simulink model "spart_sim_test"  (R2022a)
settings: Solver=VariableStepAuto  StartTime=0.0  StopTime=10.0  RelTol=1e-3
undefined symbols (not defined in the file or in its folder): M0, um0
libraries: SPART_Lib x3
settings Model: Creator=charl  LastModifiedBy=charl

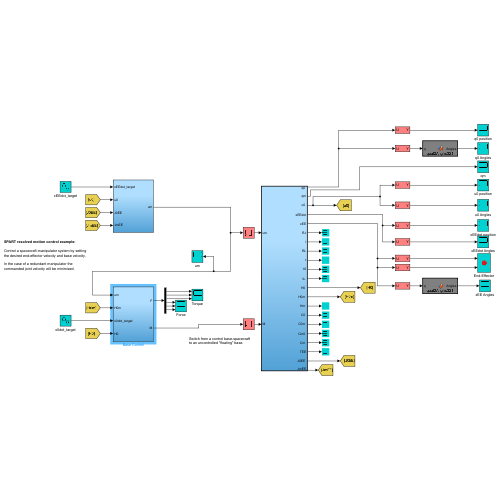
[thumbnail: Simulink's stored preview of the top-level diagram]
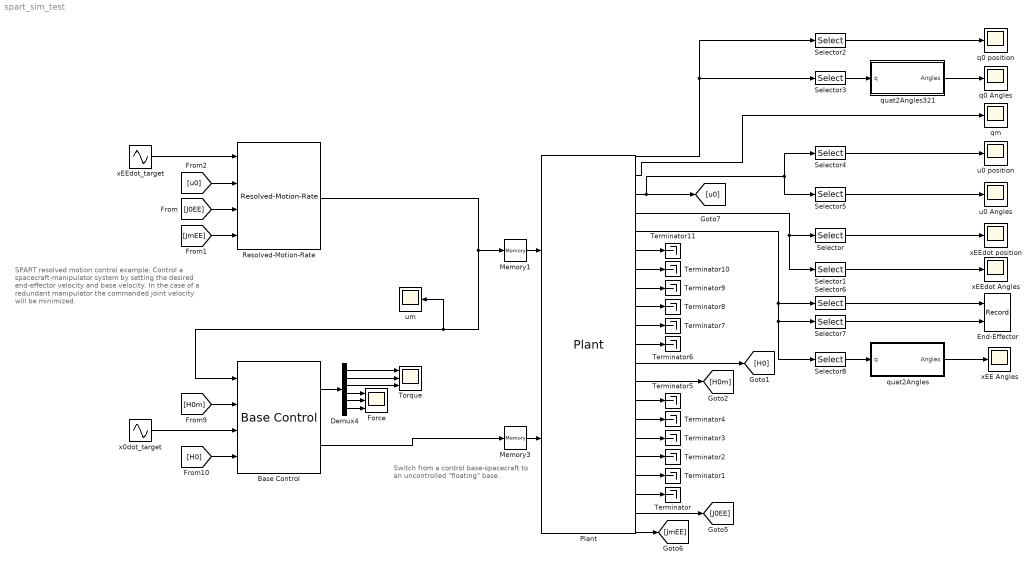
== system spart_sim_test ==
  note: SPART resolved motion control example:
      |
      | Control a spacecraft-manipulator system by setting the desired end-effector velocity and base velocity.
      |
      | In the case of a redundant manipulator the commanded joint velocity will be minimized.
  note: Switch from a control base-spacecraft to an uncontrolled "floating" base.
  Base Control : SPART_Lib/Control/Base Control  SystemSampleTime=-1  VariantActivationTime=update diagram  Latency=0  AutoFrameSizeCalculation=off
  Demux4 : Demux  Outputs=6
  End-Effector : Record  FileSettingsInternal="{\"entries\":[{\"content\":{\"excelSettings\":{\"content\":{},\"type\":\"Streamout.ExcelSettings\"}},\"type\":\"Streamout.FileSettingStorage\",\"uuid\":\"04699d78-4616-4cef-81af-d9585e3b4ee2\"}],\"packageUris\":[\"http://schema.mathworks.com/mf0/streamout_blocks/R2020a\"],\"version\":\"1.0\"}"  Layout=[1 1]  SignalsInternal="{\"entries\":[{\"content\":{\"signals\":[{\"content\":{\"blockPath\":[\"spart_sim_test/End-Effector\"],\"channel\":[],\"dimensions\":[1,1],\"domain\":\"spart_sim_test/End-Effector\",\"lineColor\":\"#a2142f\",\"plots\":[1],\"port\":1,\"sid\":[\"\"],\"signalID\":227,\"signalName\":\"Selector6\"},\"type\":\"RecordBlkView.Signal\",\"uuid\":\"8d9be762-1d05-4863-8dca-644fe018a486\"},{\"content\":{\"blockPath\":[\"spart_sim_test/End-Effector\"],\"channel\":[],\"dimensions\":[1,1],\"domain\":\"spart_sim_test/End-Effector\",\"lineColor\":\"#139fff\",\"plots\":[1],\"port\":2,\"sid\":[\"\"],\"signalID\":231,\"signalName\":\"Selector7\"},\"type\":\"RecordBlkView.Signal\",\"uuid\":\"098425a8-9d72-4562-8d53-08ba24e55e97\"}]},\"type\":\"RecordBlkView.InputSignals\",\"uuid\":\"7cb01df9-89e0-49c5-adc4-e9907efb910e\"}],\"packageUris\":[\"http://schema.mathworks.com/mf0/streamout_blocks/R2020a\"],\"version\":\"1.0\"}"  VisualizationBindings="{\"xyplotplugin\":{\"info\":[{\"series\":[{\"bindingParametersList\":[{\"parameter\":\"X-Axis\",\"signalID\":227,\"signalName\":\"Selector6\"},{\"parameter\":\"Y-Axis\",\"signalID\":231,\"signalName\":\"Selector7\"}],\"seriesID\":21343}],\"subplotID\":1}]}}"  CompatibilityTag=XY  st=-1
  Force : Scope  NumInputPorts=3
  Memory1 : Memory  InitialCondition=um0  InheritSampleTime=on
  Memory3 : Memory  InitialCondition=M0  InheritSampleTime=on
  Plant : SPART_Lib/Plant  SystemSampleTime=-1  VariantActivationTime=update diagram  Latency=0  AutoFrameSizeCalculation=off
  "Resolved-Motion-Rate " : SPART_Lib/Control/Resolved-Motion-Rate   SystemSampleTime=-1  VariantActivationTime=update diagram  Latency=0  AutoFrameSizeCalculation=off
  Selector : Selector  InputPortWidth=6  IndexOptions=Index vector (dialog)  Indices=[4:6]  OutputSizes=1
  Selector1 : Selector  InputPortWidth=6  IndexOptions=Index vector (dialog)  Indices=[1:3]  OutputSizes=1
  Selector2 : Selector  InputPortWidth=7  IndexOptions=Index vector (dialog)  Indices=[5:7]  OutputSizes=1
  Selector3 : Selector  InputPortWidth=7  IndexOptions=Index vector (dialog)  Indices=[1:4]  OutputSizes=1
  Selector4 : Selector  InputPortWidth=6  IndexOptions=Index vector (dialog)  Indices=[4:6]  OutputSizes=1
  Selector5 : Selector  InputPortWidth=6  IndexOptions=Index vector (dialog)  Indices=[1:3]  OutputSizes=1
  Selector6 : Selector  InputPortWidth=7  IndexOptions=Index vector (dialog)  Indices=[5]  OutputSizes=1
  Selector7 : Selector  InputPortWidth=7  IndexOptions=Index vector (dialog)  Indices=[6]  OutputSizes=1
  Selector8 : Selector  InputPortWidth=7  IndexOptions=Index vector (dialog)  Indices=[1:4]  OutputSizes=1
  Terminator{,1..11} (12 alike) : Terminator
  Torque : Scope  NumInputPorts=3
  q0 Angles : Scope
  "q0 position " : Scope
  qm : Scope
  quat2Angles : MATLAB Function  TreatAsAtomicUnit=on
  quat2Angles321 : MATLAB Function  TreatAsAtomicUnit=on
  u0 Angles : Scope
  u0 position : Scope
  um : Scope
  x0dot_target : Sin  Amplitude=[0;0;0.05;0;0;0]  Frequency=pi/4  SampleTime=0
  xEE Angles : Scope
  xEEdot Angles : Scope
  xEEdot position : Scope
  xEEdot_target : Sin  Amplitude=[0;0;0.1;0.05;0.05;0]  Frequency=pi/2  Phase=[0;0;0;0;pi/2;0]  SampleTime=0
  wires:
  Plant/21 -> [JmEE]
  Selector1/1 -> xEEdot Angles/1
  Plant/9 -> Terminator8/1
  Memory1/1 -> Plant/1
  Base Control/2 -> Memory3/1
  [H0] -> Base Control/4
  Memory3/1 -> Plant/2
  Plant/16 -> Terminator3/1
  quat2Angles321/1(Angles) -> q0 Angles/1
  Selector3/1 -> quat2Angles321/1(q)
  [J0EE] -> "Resolved-Motion-Rate "/3
  Plant/19 -> Terminator/1
  Selector7/1 -> End-Effector/2
  Selector6/1 -> End-Effector/1
  "Resolved-Motion-Rate "/1 -> Base Control/1, um/1, Memory1/1
  Selector4/1 -> u0 position/1
  Selector/1 -> xEEdot position/1
  Plant/1 -> Selector2/1, Selector3/1
  Plant/14 -> Terminator5/1
  Plant/11 -> Terminator6/1
  Plant/10 -> Terminator7/1
  Selector8/1 -> quat2Angles/1(q)
  Plant/8 -> Terminator9/1
  Plant/5 -> Selector6/1, Selector7/1, Selector8/1
  Selector2/1 -> "q0 position "/1
  quat2Angles/1(Angles) -> xEE Angles/1
  Plant/4 -> Selector1/1, Selector/1
  Demux4/5 -> Force/2
  Demux4/3 -> Torque/3
  Plant/7 -> Terminator10/1
  Demux4/6 -> Force/3
  Demux4/1 -> Torque/1
  Plant/15 -> Terminator4/1
  Base Control/1 -> Demux4/1
  Plant/17 -> Terminator2/1
  [u0] -> "Resolved-Motion-Rate "/2
  Plant/3 -> Selector4/1, Selector5/1, [u0]
  Demux4/4 -> Force/1
  Plant/6 -> Terminator11/1
  x0dot_target/1 -> Base Control/3
  Plant/20 -> [J0EE]
  Demux4/2 -> Torque/2
  [H0m] -> Base Control/2
  xEEdot_target/1 -> "Resolved-Motion-Rate "/1
  [JmEE] -> "Resolved-Motion-Rate "/4
  Selector5/1 -> u0 Angles/1
  Plant/12 -> [H0]
  Plant/2 -> qm/1
  Plant/13 -> [H0m]
  Plant/18 -> Terminator1/1

== matlab function spart_sim_test/quat2Angles321 ==
  data: q input; Angles output
function Angles = quat2Angles321(q)
%Convert the quaternion to Euler angles (321 sequence), x-phi, y-theta, z-psi.
%
%Uses the functions under the Utilities folder


Angles = quat_Angles321(q);

end

== matlab function spart_sim_test/quat2Angles ==
  data: q input; Angles output
function Angles = quat2Angles321(q)
%Convert the quaternion to Euler angles (321 sequence), x-phi, y-theta, z-psi.
%
%Uses the functions under the Utilities folder


Angles = quat_Angles321(q);

end
